simulink model "hybrid_dsm_adc"  (R2025b)
settings: Solver=FixedStepAuto  StartTime=0.0  StopTime=5  RelTol=1e-3
undefined symbols (not defined in the file): dspblkCoreblockFVToolHelper, gcbh
libraries: dspsigops x1
settings Model: Creator=Aman Mittal  LastModifiedBy=ashaydwivedi

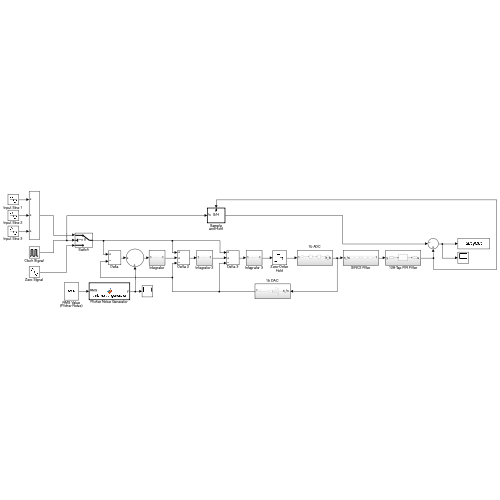
[thumbnail: Simulink's stored preview of the top-level diagram]
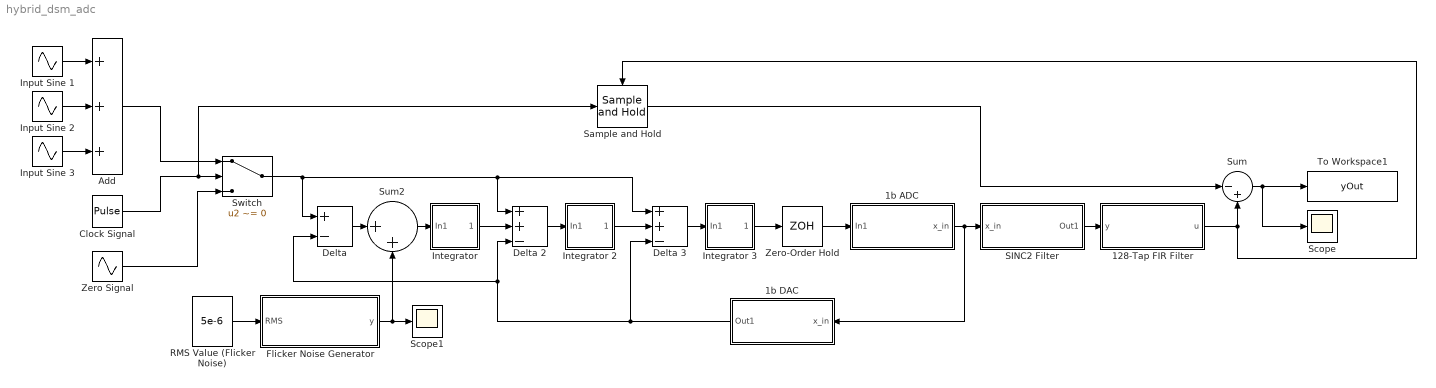
== system hybrid_dsm_adc ==
  128-Tap FIR Filter : Subsystem
  1b ADC : Subsystem
  1b DAC : Subsystem
  Add : Sum  Inputs=+++
  Clock Signal : DiscretePulseGenerator  PulseType=Time based  Period=1/100000  PulseWidth=40%
  Delta : Sum  Inputs=+-
  Delta 2 : Sum  Inputs=++-
  Delta 3 : Sum  Inputs=++-
  Flicker Noise Generator : MATLAB Function  TreatAsAtomicUnit=on
  Input Sine 1 : Sin  Amplitude=2  Frequency=2*pi*40  SampleTime=0
  Input Sine 2 : Sin  Amplitude=1.5  Frequency=2*pi*320  SampleTime=0
  Input Sine 3 : Sin  Frequency=2*pi*640  SampleTime=0
  Integrator : Subsystem
  Integrator 2 : Subsystem
  Integrator 3 : Subsystem
  RMS Value (Flicker Noise) : Constant  Value=5e-6
  SINC2 Filter : Subsystem
  Sample and Hold : dspsigops/Sample and Hold  trig=Rising edge  initCond=0  latchinput=off
  Scope : Scope
      settings: ActiveDisplayYMinimum=-24592.291708378718  ActiveDisplayYMaximum=28172.696799117439
  Scope1 : Scope
      settings: ActiveDisplayYMinimum=-8.1562596531748737E-5  ActiveDisplayYMaximum=8.0150088014313336E-5
  Sum : Sum  Inputs=|-+
  Sum2 : Sum  Inputs=|++
  Switch : Switch  Criteria=u2 ~= 0  SaturateOnIntegerOverflow=off  InputSameDT=off
  To Workspace1 : ToWorkspace  VariableName=yOut  SaveFormat=Timeseries  SampleTime=-1
  Zero Signal : Sin  Amplitude=0.0  Frequency=2*pi*20  SampleTime=0
  Zero-Order Hold : ZeroOrderHold  SampleTime=(1/2000)*(1/1025)
  wires:
  Delta/1 -> Sum2/1
  Input Sine 2/1 -> Add/2
  SINC2 Filter/1(Out1) -> 128-Tap FIR Filter/1(y)
  Delta 2/1 -> Integrator 2/1(In1)
  Switch/1 -> Delta/1, Delta 3/1, Delta 2/1
  Input Sine 1/1 -> Add/1
  Input Sine 3/1 -> Add/3
  Flicker Noise Generator/1(y) -> Sum2/2, Scope1/1
  Sample and Hold/1 -> Sum/1
  Clock Signal/1 -> Sample and Hold/1, Switch/2
  RMS Value (Flicker Noise)/1 -> Flicker Noise Generator/1(RMS)
  1b DAC/1(Out1) -> Delta 3/3, Delta 2/3, Delta/2
  Zero Signal/1 -> Switch/3
  1b ADC/1(x_in) -> SINC2 Filter/1(x_in), 1b DAC/1(x_in)
  Delta 3/1 -> Integrator 3/1(In1)
  Sum2/1 -> Integrator/1(In1)
  Sum/1 -> Scope/1, To Workspace1/1
  Integrator/1(Out1) -> Delta 2/2
  Add/1 -> Switch/1
  128-Tap FIR Filter/1(u) -> Sum/2, Sample and Hold/Trigger
  Integrator 2/1(Out1) -> Delta 3/2
  Integrator 3/1(Out1) -> Zero-Order Hold/1
  Zero-Order Hold/1 -> 1b ADC/1(In1)

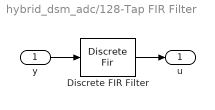
== system hybrid_dsm_adc/128-Tap FIR Filter ==
  y : Inport
  Discrete FIR Filter : DiscreteFir  LoadFcn=dspblkCoreblockFVToolHelper(gcbh,'load');  Coefficients=[0.0078125 0.0078125 0.0078125 0.0078125 0.0078125 0.0078125 0.0078125 0.0078125 0.0078125 0.0078125 0.0078125 0.0078125 0.0078125 0.0078125 0.0078125 0.0078125 0.0078125 0.0078125 0.0078125 0.0078125 0.0078125 0.0078125 0.0078125 0.0078125 0.0078125 0.0078125 0.0078125 0.0078125 0.0078125 0.0078125 0.0078125 0.0078125 0.0078125 0.0078125 0.0078125 0.0078125 0.0078125 0.0078125 0.0078125 0.0078125 0.0078125 0.0078125 0.0078125 0.0078125 0.0078125 0.0078125 0.0078125 0.0078125 0.0078125 0.0078125 0.0078125 0.0078125 0.0078125 0.0078125 0.0078125 0.0078125 0.0078125 0.0078125 0.0078125 0.0078125 0.0078125 0.0078125 0.0078125 0.0078125 0.0078125 0.0078125 0.0078125 0.0078125 0.0078125 0.0078125 0.0078125 0.0078125 0.0078125 0.0078125 0.0078125 0.0078125 0.0078125 0.0078125 0.0078125 0.0078125 0.0078125 0.0078125 0.0078125 0.0078125 0.0078125 0.0078125 0.0078125 0.0078125 0.0078125 0.0078125 0.0078125 0.0078125 0.0078125 0.0078125 0.0078125 0.0078125 0.0078125 0.0078125 0.0078125 0.0078125 0.0078125 0.0078125 0.0078125 0.0078125 0.0078125 0.0078125 0.0078125 0.0078125 0.0078125 0.0078125 0.0078125 0.0078125 0.0078125 0.0078125 0.0078125 0.0078125 0.0078125 0.0078125 0.0078125 0.0078125 0.0078125 0.0078125 0.0078125 0.0078125 0.0078125 0.0078125 0.0078125 0.0078125 0.0078125 0.0078125 0.0078125 0.0078125 0.0078125 0.0078125 0.0078125 0.0078125]
      settings: CopyFcn=dspblkCoreblockFVToolHelper(gcbh,'copy');  DeleteFcn=dspblkCoreblockFVToolHelper(gcbh,'close');  ModelCloseFcn=dspblkCoreblockFVToolHelper(gcbh,'close');  PreSaveFcn=dspblkCoreblockFVToolHelper(gcbh,'presave');  PostSaveFcn=dspblkCoreblockFVToolHelper(gcbh,'postsave');  CloseFcn=dspblkCoreblockFVToolHelper(gcbh,'close');
  u : Outport
  wires:
  y/1 -> Discrete FIR Filter/1
  Discrete FIR Filter/1 -> u/1

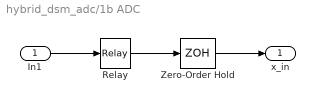
== system hybrid_dsm_adc/1b ADC ==
  In1 : Inport
  Relay : Relay  OnSwitchValue=0  OffSwitchValue=0  OffOutputValue=-1  ZeroCross=off
  Zero-Order Hold : ZeroOrderHold  SampleTime=(1/2000)*(1/1025)
  x_in : Outport
  wires:
  In1/1 -> Relay/1
  Relay/1 -> Zero-Order Hold/1
  Zero-Order Hold/1 -> x_in/1

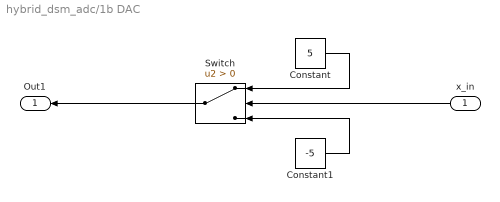
== system hybrid_dsm_adc/1b DAC ==
  x_in : Inport
  Constant : Constant  Value=5
  Constant1 : Constant  Value=-5
  Switch : Switch  Criteria=u2 > Threshold  SaturateOnIntegerOverflow=off  InputSameDT=off
  Out1 : Outport
  wires:
  x_in/1 -> Switch/2
  Constant/1 -> Switch/1
  Constant1/1 -> Switch/3
  Switch/1 -> Out1/1

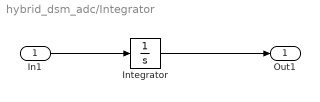
== system hybrid_dsm_adc/Integrator ==
  In1 : Inport
  Integrator : Integrator
  Out1 : Outport
  wires:
  In1/1 -> Integrator/1
  Integrator/1 -> Out1/1

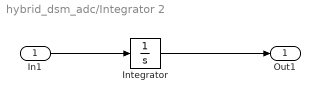
== system hybrid_dsm_adc/Integrator 2 ==
  In1 : Inport
  Integrator : Integrator
  Out1 : Outport
  wires:
  In1/1 -> Integrator/1
  Integrator/1 -> Out1/1

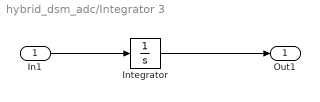
== system hybrid_dsm_adc/Integrator 3 ==
  In1 : Inport
  Integrator : Integrator
  Out1 : Outport
  wires:
  In1/1 -> Integrator/1
  Integrator/1 -> Out1/1

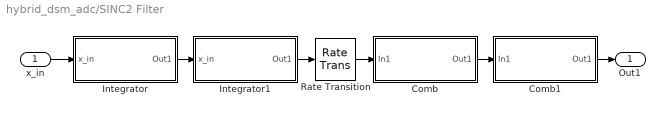
== system hybrid_dsm_adc/SINC2 Filter ==
  x_in : Inport
  Comb : Subsystem
  Comb1 : Subsystem
  Integrator : Subsystem
  Integrator1 : Subsystem
  Rate Transition : RateTransition  OutPortSampleTime=1/2000
  Out1 : Outport
  wires:
  x_in/1 -> Integrator/1(x_in)
  Rate Transition/1 -> Comb/1(In1)
  Integrator/1(Out1) -> Integrator1/1(x_in)
  Integrator1/1(Out1) -> Rate Transition/1
  Comb/1(Out1) -> Comb1/1(In1)
  Comb1/1(Out1) -> Out1/1

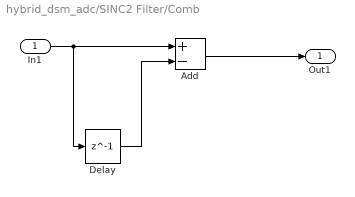
== system hybrid_dsm_adc/SINC2 Filter/Comb ==
  In1 : Inport
  Add : Sum  Inputs=+-
  Delay : Delay  DelayLength=1  InitialCondition=0
  Out1 : Outport
  wires:
  In1/1 -> Delay/1, Add/1
  Add/1 -> Out1/1
  Delay/1 -> Add/2

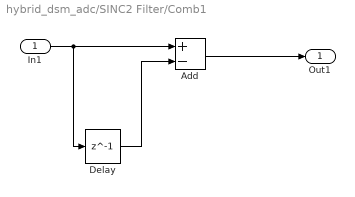
== system hybrid_dsm_adc/SINC2 Filter/Comb1 ==
  In1 : Inport
  Add : Sum  Inputs=+-
  Delay : Delay  DelayLength=1  InitialCondition=0
  Out1 : Outport
  wires:
  In1/1 -> Delay/1, Add/1
  Add/1 -> Out1/1
  Delay/1 -> Add/2

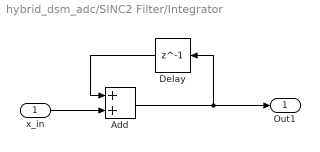
== system hybrid_dsm_adc/SINC2 Filter/Integrator ==
  x_in : Inport
  Add : Sum
  Delay : Delay  DelayLength=1  InitialCondition=0
  Out1 : Outport
  wires:
  x_in/1 -> Add/2
  Add/1 -> Delay/1, Out1/1
  Delay/1 -> Add/1

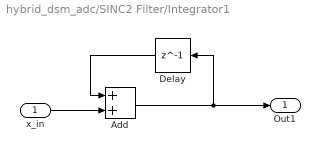
== system hybrid_dsm_adc/SINC2 Filter/Integrator1 ==
  x_in : Inport
  Add : Sum
  Delay : Delay  DelayLength=1  InitialCondition=0
  Out1 : Outport
  wires:
  x_in/1 -> Add/2
  Add/1 -> Delay/1, Out1/1
  Delay/1 -> Add/1

== matlab function hybrid_dsm_adc/Flicker Noise Generator ==
  data: y output; RMS input
function y = pink_noise_generator(RMS)
    % Generator Parameters
    tau = [1e-4, 1e-3, 1e-2, 1e-1];   
    alpha = [0.185, 0.27, 0.24, 0.15];  
    V_RMS_TARGET = RMS;
    RMS_UNSCALED_NOISE = 43.5;
    G_scale = V_RMS_TARGET / RMS_UNSCALED_NOISE;

    persistent x Ts_cached

    if isempty(x)
        x = zeros(4,1);
    end
    
    if isempty(Ts_cached)
        Ts_cached = 1e-6; % Sampling Time
    end
    Ts = Ts_cached;

    % Loop to Generate Noise
    w = randn;   
    y_sum = 0;
    for k = 1:4
        a = exp(-Ts / tau(k));           
        x(k) = a * x(k) + alpha(k) * w;
        y_sum = y_sum + x(k);
    end
    
    % Display Output
    y = y_sum * G_scale;
end
